simulink model "symulacja_dyskretny"  (R2013a)
settings: Solver=ode45  SolverMode=SingleTasking  StartTime=0.0  StopTime=20  RelTol=1e-3
values from neighbouring files (symbols this model uses):
  J = 22*Js    (= 6.05)    [dane.m]
  Kp = 1.5*Un/10    (= 33)    [dane.m]
  Kt = 10/(1.2*wn)    (= 0.0530516476973)    [dane.m]
  Mn = psi_n*In    [dane.m]
  psi_e = (Un-In*R)/wn    (= 1.31652968926)    [dane.m]
  Rt = 0.15    [dane.m]
  T = L/R    (= 0.125)    [dane.m]
  Un = 220    [dane.m]
  wn = 2*pi*nn/60    (= 157.079632679)    [dane.m]
  Y = 10/(2.5*In)    (= 0.0454545454545)    [dane.m]
undefined symbols (not defined in the file or in its folder): K1, K2, K3, K4, Tp, Uz0
libraries: powerlib x1
settings Model: Creator=user  LastModifiedBy=Wojciech
settings DataIOCC: SignalLoggingSaveFormat=ModelDataLogs
settings OptimizationCC: BlockReduction=off  BooleanDataType=off
settings DebuggingCC: SaveWithParameterizedLinksMsg=none  SignalResolutionControl=TryResolveAllWithWarning  SolverPrmCheckMsg=none  MultiTaskDSMMsg=warning  MultiTaskCondExecSysMsg=none  StrictBusMsg=None
settings HardwareCC: TargetUnknown=on
settings RTWCC: IncludeERTFirstTime=on

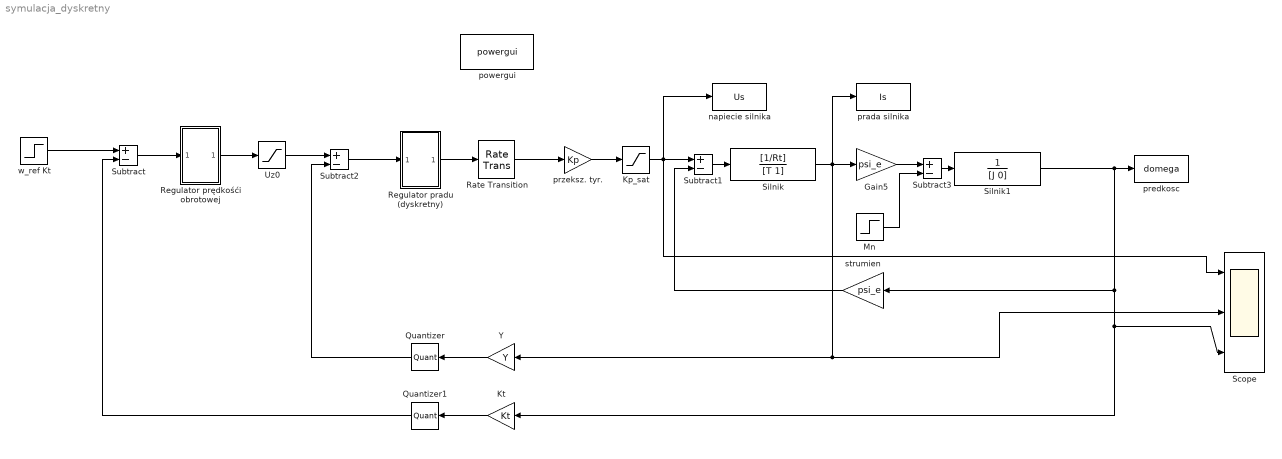
== system symulacja_dyskretny ==
  Gain5 : Gain  Gain=psi_e
  Kp_sat : Saturate  UpperLimit=1.5*Un  LowerLimit=-1.5*Un
  Kt : Gain  Gain=Kt
  Mn : Step  Time=0  After=Mn  SampleTime=0
  Quantizer : Quantizer  QuantizationInterval=10/4095
  Quantizer1 : Quantizer  QuantizationInterval=10/4095
  Rate Transition : RateTransition  OutPortSampleTime=Tp
  Regulator pradu (dyskretny) : Subsystem
  Regulator prędkośći obrotowej : Subsystem
  Scope : Scope  NumInputPorts=3
      settings: YMin=-5~-5~-5  YMax=5~5~5
  Silnik : TransferFcn  Numerator=[1/Rt]  Denominator=[T 1]
  Silnik1 : TransferFcn  Numerator=1  Denominator=[J 0]
  Subtract{,1..3} (4 alike) : Sum  Inputs=+-
  Uz0 : Saturate  UpperLimit=Uz0  LowerLimit=-Uz0
  Y : Gain  Gain=Y
  napiecie silnika : ToWorkspace  VariableName=Us  SampleTime=-1  SaveFormat=Structure With Time
  powergui : powerlib/powergui  Priority=1  SimulationMode=Continuous  SolverType=Tustin  SampleTime=50e-6  frequency=60  SPID=off  DisableSnubberDevices=off  DisableRonSwitches=off  DisableVfSwitches=off  SwTol=0  Interpol=off  DisplayEquations=off  frequencyindice=60  Pbase=100e6  ErrMax=1e-4  Iterations=50  UnitsV=kV  UnitsW=MW  FunctionMessages=off  echomessages=off  HookPort=off  EnableUseOfTLC=off  x0status=blocks  RestoreLinks=warning  ResistiveCurrentMeasurement=off  Frange=[0:2:500]  Ylog=off  Xlog=on  ShowGrid=off  save=off  variable=ZData  ZoomFFT=off  StartTime=0.0  cycles=1  DisplayStyle=1  fundamental=60  FreqAxis=off  MaxFrequency=1000  frequencyindicesteady=1  RmsSteady=1  display=off  Ts=0  methode=off
  prada silnika : ToWorkspace  VariableName=Is  SampleTime=-1  SaveFormat=Structure With Time
  predkosc : ToWorkspace  VariableName=domega  SampleTime=-1  SaveFormat=Timeseries
  przeksz. tyr. : Gain  Gain=Kp
  strumien : Gain  Gain=psi_e
  w_ref Kt : Step  Time=0  Before=wn*Kt  After=wn*Kt  SampleTime=Tp
  wires:
  przeksz. tyr./1 -> Kp_sat/1
  Subtract1/1 -> Silnik/1
  Silnik/1 -> prada silnika/1, Scope/2, Y/1, Gain5/1
  Gain5/1 -> Subtract3/1
  Subtract3/1 -> Silnik1/1
  Mn/1 -> Subtract3/2
  strumien/1 -> Subtract1/2
  Kp_sat/1 -> Scope/1, napiecie silnika/1, Subtract1/1
  Uz0/1 -> Subtract2/1
  Silnik1/1 -> predkosc/1, strumien/1, Kt/1, Scope/3
  w_ref Kt/1 -> Subtract/1
  Kt/1 -> Quantizer1/1
  Quantizer1/1 -> Subtract/2
  Subtract2/1 -> Regulator pradu (dyskretny)/1(In1)
  Regulator prędkośći obrotowej/1(Out1) -> Uz0/1
  Subtract/1 -> Regulator prędkośći obrotowej/1(In1)
  Y/1 -> Quantizer/1
  Quantizer/1 -> Subtract2/2
  Regulator pradu (dyskretny)/1(Out1) -> Rate Transition/1
  Rate Transition/1 -> przeksz. tyr./1

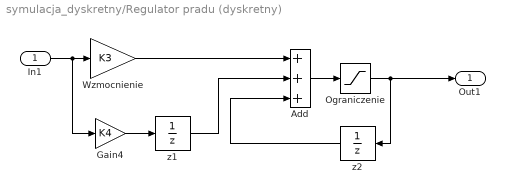
== system symulacja_dyskretny/Regulator pradu (dyskretny) ==
  In1 : Inport
  Add : Sum  Inputs=+++
  Gain4 : Gain  Gain=K4
  Ograniczenie : Saturate  UpperLimit=10  LowerLimit=-10
  Wzmocnienie : Gain  Gain=K3
  z1 : UnitDelay  SampleTime=-1
  z2 : UnitDelay  SampleTime=-1
  Out1 : Outport
  wires:
  In1/1 -> Gain4/1, Wzmocnienie/1
  Wzmocnienie/1 -> Add/1
  Gain4/1 -> z1/1
  z1/1 -> Add/2
  Add/1 -> Ograniczenie/1
  Ograniczenie/1 -> Out1/1, z2/1
  z2/1 -> Add/3

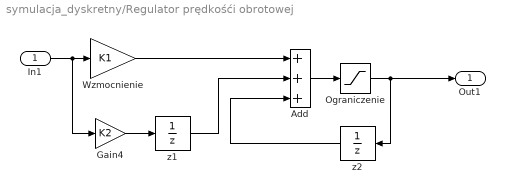
== system symulacja_dyskretny/Regulator prędkośći obrotowej ==
  In1 : Inport
  Add : Sum  Inputs=+++
  Gain4 : Gain  Gain=K2
  Ograniczenie : Saturate  UpperLimit=10  LowerLimit=-10
  Wzmocnienie : Gain  Gain=K1
  z1 : UnitDelay  SampleTime=Tp
  z2 : UnitDelay  SampleTime=Tp
  Out1 : Outport
  wires:
  In1/1 -> Gain4/1, Wzmocnienie/1
  Wzmocnienie/1 -> Add/1
  Gain4/1 -> z1/1
  z1/1 -> Add/2
  Add/1 -> Ograniczenie/1
  Ograniczenie/1 -> Out1/1, z2/1
  z2/1 -> Add/3
